simulink model "Hierarchical_control"  (R2023a)
settings: Solver=VariableStepAuto  StartTime=0.0  StopTime=T  RelTol=1e-3
InitFcn:
  | %% INITIALIZATION
  | run('LOAD_HIERARCHICAL.m');
  | %% UAV PARAMETERS
  | mass = 0.85;
  | Ib = diag([2.5 2.1 4.3])*10^-2;
  | %% SAMPLING TIME
  | Ts=0.01;
libraries: robotcorelib x1, uavutilslib x1
settings Model: Creator=salvatoregranata  LastModifiedBy=salvatoregranata

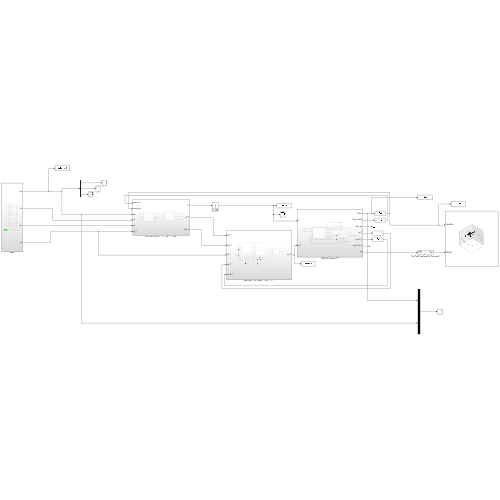
[thumbnail: Simulink's stored preview of the top-level diagram]
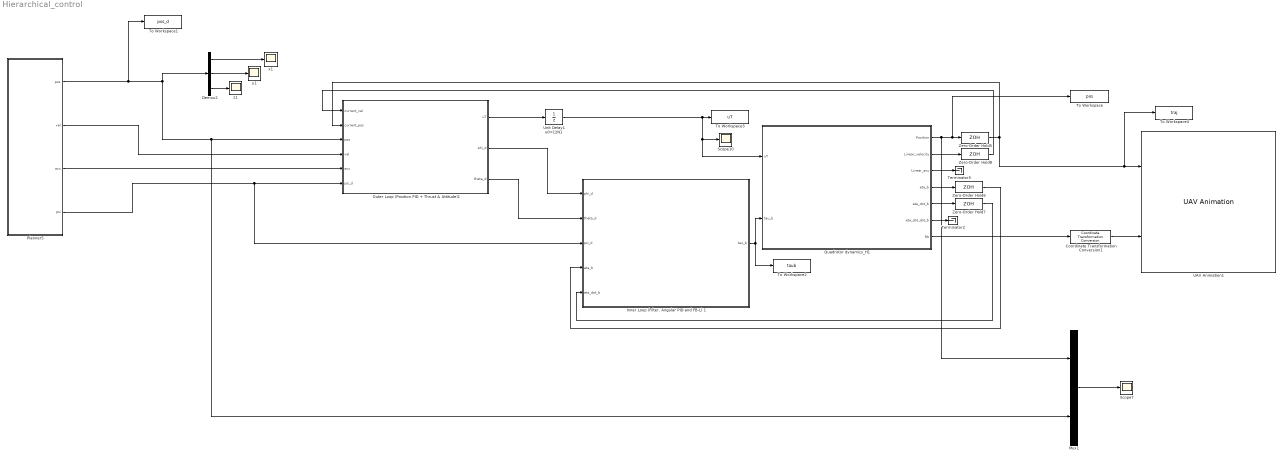
== system Hierarchical_control ==
  Coordinate Transformation Conversion1 : robotcorelib/Coordinate Transformation Conversion  InputRepresentation=Rotation Matrix  InputEulerSequence=ZYX  ShowTrVecInputPort=on  OutputRepresentation=Quaternion  OutputEulerSequence=ZYX  ShowTrVecOutputPort=on  SimulateUsing=Interpreted execution
  Demux2 : Demux  Outputs=3
  "Inner Loop (Filter, Angular PID and FB-L) 1" : Subsystem
  Mux1 : Mux  Inputs=2
  Outer Loop (Position PID + Thrust & Attitude)1 : Subsystem
  Planner5 : Subsystem
  Quadrotor dynamics_H1 : Subsystem
  Scope10 : Scope
  Scope7 : Scope
  Terminator2 : Terminator
  Terminator5 : Terminator
  To Workspace : ToWorkspace  VariableName=pos  SaveFormat=Structure With Time  SampleTime=-1
  To Workspace1 : ToWorkspace  VariableName=pos_d  SaveFormat=Structure With Time  SampleTime=-1
  To Workspace2 : ToWorkspace  VariableName=taub  SaveFormat=Structure With Time  SampleTime=-1
  To Workspace3 : ToWorkspace  VariableName=uT  SaveFormat=Structure With Time  SampleTime=-1
  To Workspace4 : ToWorkspace  VariableName=traj  SaveFormat=Structure With Time  SampleTime=-1
  UAV Animation1 : uavutilslib/UAV Animation  UAVType=Multirotor  UAVSize=1  InertialZDirection=Up  SampleTime=0.001
  Unit Delay1 u0=12N1 : UnitDelay  InitialCondition=11.772  SampleTime=Ts
  Zero-Order Hold{5..8} (4 alike) : ZeroOrderHold  SampleTime=Ts
  x1 : Scope
  y1 : Scope
  z1 : Scope
  wires:
  Coordinate Transformation Conversion1/1 -> UAV Animation1/2
  Quadrotor dynamics_H1/5(eta_dot_b) -> Zero-Order Hold7/1
  "Inner Loop (Filter, Angular PID and FB-L) 1"/1(tau_b) -> To Workspace2/1, Quadrotor dynamics_H1/2(tau_b)
  Planner5/3(acc) -> Outer Loop (Position PID + Thrust & Attitude)1/5(acc)
  Quadrotor dynamics_H1/6(eta_dot_dot_b) -> Terminator2/1
  Quadrotor dynamics_H1/2(Linear_velocity) -> Zero-Order Hold8/1
  Zero-Order Hold8/1 -> Outer Loop (Position PID + Thrust & Attitude)1/1(current_vel)
  Planner5/1(pos) -> To Workspace1/1, Mux1/2, Outer Loop (Position PID + Thrust & Attitude)1/3(pos), Demux2/1
  Mux1/1 -> Scope7/1
  Zero-Order Hold6/1 -> "Inner Loop (Filter, Angular PID and FB-L) 1"/4(eta_b)
  Outer Loop (Position PID + Thrust & Attitude)1/1(uT) -> Unit Delay1 u0=12N1/1
  Demux2/1 -> x1/1
  Zero-Order Hold7/1 -> "Inner Loop (Filter, Angular PID and FB-L) 1"/5(eta_dot_b)
  Planner5/4(psi) -> "Inner Loop (Filter, Angular PID and FB-L) 1"/3(psi_d), Outer Loop (Position PID + Thrust & Attitude)1/6(psi_d)
  Unit Delay1 u0=12N1/1 -> To Workspace3/1, Scope10/1, Quadrotor dynamics_H1/1(uT)
  Demux2/3 -> z1/1
  Demux2/2 -> y1/1
  Outer Loop (Position PID + Thrust & Attitude)1/3(theta_d) -> "Inner Loop (Filter, Angular PID and FB-L) 1"/2(theta_d)
  Quadrotor dynamics_H1/7(Rb) -> Coordinate Transformation Conversion1/1
  Quadrotor dynamics_H1/4(eta_b) -> Zero-Order Hold6/1
  Outer Loop (Position PID + Thrust & Attitude)1/2(phi_d) -> "Inner Loop (Filter, Angular PID and FB-L) 1"/1(phi_d)
  Quadrotor dynamics_H1/1(Position) -> Mux1/1, To Workspace/1, Zero-Order Hold5/1
  Quadrotor dynamics_H1/3(Linear_acc) -> Terminator5/1
  Planner5/2(vel) -> Outer Loop (Position PID + Thrust & Attitude)1/4(vel)
  Zero-Order Hold5/1 -> To Workspace4/1, UAV Animation1/1, Outer Loop (Position PID + Thrust & Attitude)1/2(current_pos)

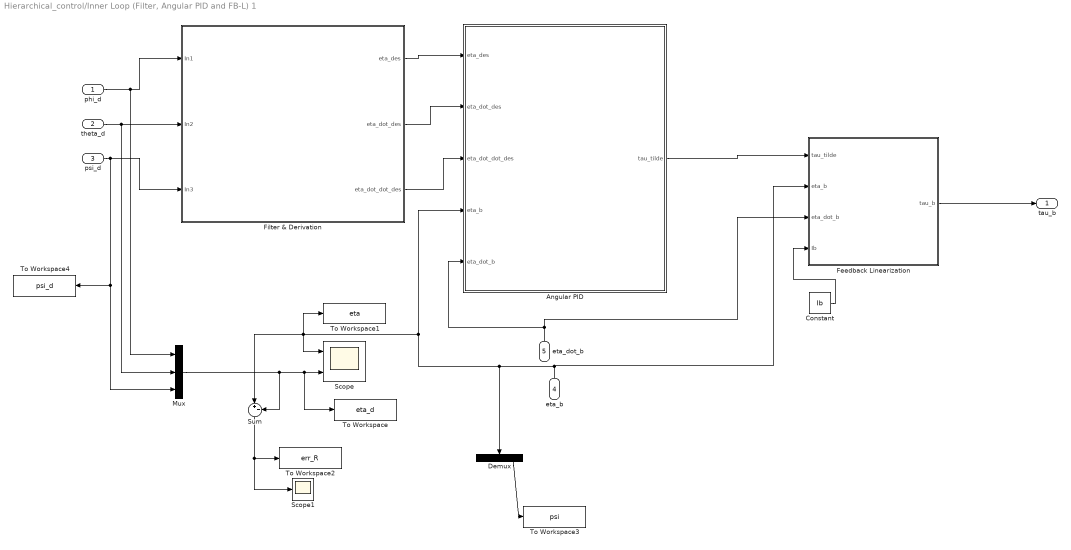
== system Hierarchical_control/Inner Loop (Filter, Angular PID and FB-L) 1 ==
  phi_d : Inport
  theta_d : Inport  Port=2
  psi_d : Inport  Port=3
  eta_b : Inport  Port=4
  eta_dot_b : Inport  Port=5
  Angular PID : MATLAB Function  TreatAsAtomicUnit=on
  Constant : Constant  Value=Ib
  Demux : Demux  Outputs=3
  Feedback Linearization : MATLAB Function  TreatAsAtomicUnit=on
  Filter & Derivation : Subsystem
  Mux : Mux  Inputs=3
  Scope : Scope  NumInputPorts=2
  Scope1 : Scope
  Sum : Sum  Inputs=|+-
  To Workspace : ToWorkspace  VariableName=eta_d  SaveFormat=Structure With Time  SampleTime=-1
  To Workspace1 : ToWorkspace  VariableName=eta  SaveFormat=Structure With Time  SampleTime=-1
  To Workspace2 : ToWorkspace  VariableName=err_R  SaveFormat=Structure With Time  SampleTime=-1
  To Workspace3 : ToWorkspace  VariableName=psi  SaveFormat=Structure With Time  SampleTime=-1
  To Workspace4 : ToWorkspace  VariableName=psi_d  SaveFormat=Structure With Time  SampleTime=-1
  tau_b : Outport
  wires:
  phi_d/1 -> Mux/1, Filter & Derivation/1(In1)
  theta_d/1 -> Mux/2, Filter & Derivation/2(In2)
  psi_d/1 -> Mux/3, To Workspace4/1, Filter & Derivation/3(In3)
  Filter & Derivation/1(eta_des) -> Angular PID/1(eta_des)
  Filter & Derivation/2(eta_dot_des) -> Angular PID/2(eta_dot_des)
  Filter & Derivation/3(eta_dot_dot_des) -> Angular PID/3(eta_dot_dot_des)
  Angular PID/1(tau_tilde) -> Feedback Linearization/1(tau_tilde)
  Feedback Linearization/1(tau_b) -> tau_b/1
  eta_b/1 -> Feedback Linearization/2(eta_b), Sum/1, Scope/1, To Workspace1/1, Angular PID/4(eta_b), Demux/1
  eta_dot_b/1 -> Angular PID/5(eta_dot_b), Feedback Linearization/3(eta_dot_b)
  Constant/1 -> Feedback Linearization/4(Ib)
  Mux/1 -> Sum/2, To Workspace/1, Scope/2
  Sum/1 -> Scope1/1, To Workspace2/1
  Demux/3 -> To Workspace3/1

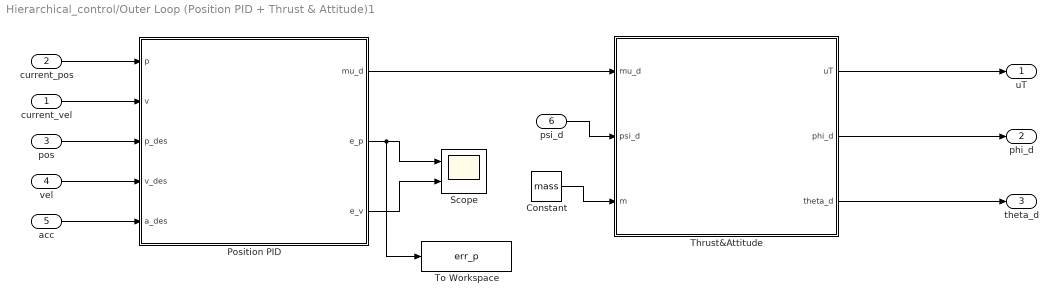
== system Hierarchical_control/Outer Loop (Position PID + Thrust & Attitude)1 ==
  current_vel : Inport
  current_pos : Inport  Port=2
  pos : Inport  Port=3
  vel : Inport  Port=4
  acc : Inport  Port=5
  psi_d : Inport  Port=6
  Constant : Constant  Value=mass
  Position PID : MATLAB Function  TreatAsAtomicUnit=on
  Scope : Scope  NumInputPorts=2
  Thrust&Attitude : MATLAB Function  TreatAsAtomicUnit=on
  To Workspace : ToWorkspace  VariableName=err_p  SaveFormat=Structure With Time  SampleTime=-1
  uT : Outport
  phi_d : Outport  Port=2
  theta_d : Outport  Port=3
  wires:
  pos/1 -> Position PID/3(p_des)
  vel/1 -> Position PID/4(v_des)
  acc/1 -> Position PID/5(a_des)
  Position PID/2(e_p) -> To Workspace/1, Scope/1
  Position PID/3(e_v) -> Scope/2
  Position PID/1(mu_d) -> Thrust&Attitude/1(mu_d)
  Thrust&Attitude/1(uT) -> uT/1
  Thrust&Attitude/2(phi_d) -> phi_d/1
  Thrust&Attitude/3(theta_d) -> theta_d/1
  psi_d/1 -> Thrust&Attitude/2(psi_d)
  current_pos/1 -> Position PID/1(p)
  current_vel/1 -> Position PID/2(v)
  Constant/1 -> Thrust&Attitude/3(m)

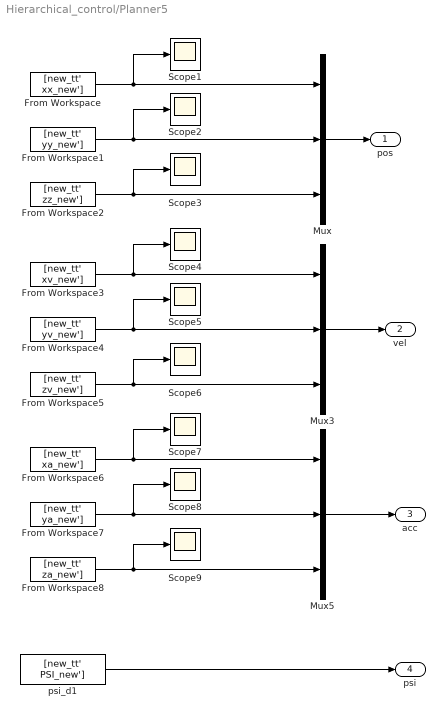
== system Hierarchical_control/Planner5 ==
  From Workspace : FromWorkspace  VariableName=[new_tt' xx_new']
  From Workspace1 : FromWorkspace  VariableName=[new_tt' yy_new']
  From Workspace2 : FromWorkspace  VariableName=[new_tt' zz_new']
  From Workspace3 : FromWorkspace  VariableName=[new_tt' xv_new']
  From Workspace4 : FromWorkspace  VariableName=[new_tt' yv_new']
  From Workspace5 : FromWorkspace  VariableName=[new_tt' zv_new']
  From Workspace6 : FromWorkspace  VariableName=[new_tt' xa_new']
  From Workspace7 : FromWorkspace  VariableName=[new_tt' ya_new']
  From Workspace8 : FromWorkspace  VariableName=[new_tt' za_new']
  Mux : Mux  Inputs=3
  Mux3 : Mux  Inputs=3
  Mux5 : Mux  Inputs=3
  Scope{1..9} (9 alike) : Scope
  psi_d1 : FromWorkspace  VariableName=[new_tt' PSI_new']  SampleTime=Ts
  pos : Outport
  vel : Outport  Port=2
  acc : Outport  Port=3
  psi : Outport  Port=4
  wires:
  Mux5/1 -> acc/1
  From Workspace1/1 -> Mux/2, Scope2/1
  Mux3/1 -> vel/1
  From Workspace6/1 -> Mux5/1, Scope7/1
  From Workspace2/1 -> Mux/3, Scope3/1
  From Workspace4/1 -> Mux3/2, Scope5/1
  Mux/1 -> pos/1
  From Workspace/1 -> Mux/1, Scope1/1
  From Workspace7/1 -> Mux5/2, Scope8/1
  From Workspace8/1 -> Scope9/1, Mux5/3
  From Workspace3/1 -> Mux3/1, Scope4/1
  From Workspace5/1 -> Mux3/3, Scope6/1
  psi_d1/1 -> psi/1

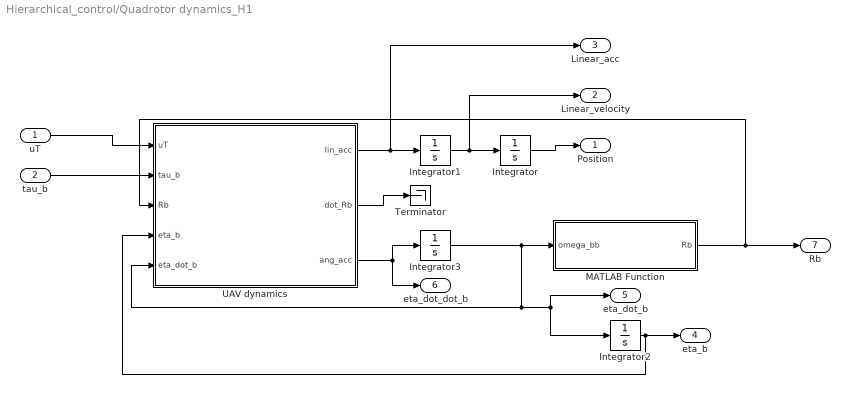
== system Hierarchical_control/Quadrotor dynamics_H1 ==
  uT : Inport
  tau_b : Inport  Port=2
  Integrator : Integrator  InitialCondition=[-1 -1.2 2]
  Integrator1 : Integrator  InitialCondition=[0 0 0]
  Integrator2 : Integrator  InitialCondition=[0 0 0]
  Integrator3 : Integrator  InitialCondition=[0 0 0]
  MATLAB Function : MATLAB Function  TreatAsAtomicUnit=on
  Terminator : Terminator
  UAV dynamics : MATLAB Function  TreatAsAtomicUnit=on
  Position : Outport
  Linear_velocity : Outport  Port=2
  Linear_acc : Outport  Port=3
  eta_b : Outport  Port=4
  eta_dot_b : Outport  Port=5
  eta_dot_dot_b : Outport  Port=6
  Rb : Outport  Port=7
  wires:
  tau_b/1 -> UAV dynamics/2(tau_b)
  Integrator/1 -> Position/1
  UAV dynamics/3(ang_acc) -> Integrator3/1, eta_dot_dot_b/1
  UAV dynamics/1(lin_acc) -> Linear_acc/1, Integrator1/1
  uT/1 -> UAV dynamics/1(uT)
  Integrator1/1 -> Linear_velocity/1, Integrator/1
  Integrator3/1 -> UAV dynamics/5(eta_dot_b), eta_dot_b/1, Integrator2/1, MATLAB Function/1(omega_bb)
  UAV dynamics/2(dot_Rb) -> Terminator/1
  MATLAB Function/1(Rb) -> Rb/1, UAV dynamics/3(Rb)
  Integrator2/1 -> UAV dynamics/4(eta_b), eta_b/1

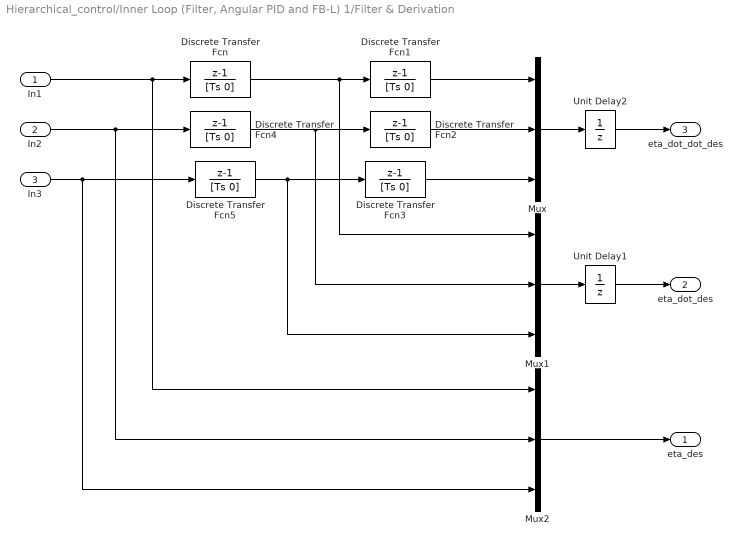
== system Hierarchical_control/Inner Loop (Filter, Angular PID and FB-L) 1/Filter & Derivation ==
  In1 : Inport
  In2 : Inport  Port=2
  In3 : Inport  Port=3
  Discrete Transfer Fcn{,1..5} (6 alike) : DiscreteTransferFcn  Numerator=[1 -1]  Denominator=[Ts 0]  SampleTime=Ts
  Mux : Mux  Inputs=3
  Mux1 : Mux  Inputs=3
  Mux2 : Mux  Inputs=3
  Unit Delay1 : UnitDelay  InitialCondition=[0 0 0]  SampleTime=Ts
  Unit Delay2 : UnitDelay  InitialCondition=[0 0 0]  SampleTime=Ts
  eta_des : Outport
  eta_dot_des : Outport  Port=2
  eta_dot_dot_des : Outport  Port=3
  wires:
  Discrete Transfer Fcn3/1 -> Mux/3
  Unit Delay1/1 -> eta_dot_des/1
  Discrete Transfer Fcn1/1 -> Mux/1
  In2/1 -> Discrete Transfer Fcn4/1, Mux2/2
  Unit Delay2/1 -> eta_dot_dot_des/1
  Discrete Transfer Fcn/1 -> Discrete Transfer Fcn1/1, Mux1/1
  Discrete Transfer Fcn2/1 -> Mux/2
  Discrete Transfer Fcn5/1 -> Mux1/3, Discrete Transfer Fcn3/1
  In3/1 -> Discrete Transfer Fcn5/1, Mux2/3
  Mux/1 -> Unit Delay2/1
  Discrete Transfer Fcn4/1 -> Discrete Transfer Fcn2/1, Mux1/2
  Mux2/1 -> eta_des/1
  Mux1/1 -> Unit Delay1/1
  In1/1 -> Discrete Transfer Fcn/1, Mux2/1

== matlab function Hierarchical_control/Inner Loop (Filter, Angular PID and FB-L) 1/Angular PID ==
  data: eta_des input; tau_tilde output; eta_dot_des input; eta_dot_dot_des input; eta_b input; eta_dot_b input
function tau_tilde = fcn(eta_des, eta_dot_des, eta_dot_dot_des, eta_b, eta_dot_b)

Ke=[diag([3 3 3]),diag([2 2 15])];

%compute the error
e_eta = eta_b-eta_des;
e_omega = eta_dot_b-eta_dot_des;
e=[e_eta;e_omega];

%simulate PD+
tau_tilde = -Ke*e + eta_dot_dot_des;

end

== matlab function Hierarchical_control/Inner Loop (Filter, Angular PID and FB-L) 1/Feedback Linearization ==
  data: tau_tilde input; tau_b output; eta_b input; eta_dot_b input; Ib input
function tau_b = fcn(tau_tilde,eta_b,eta_dot_b,Ib)

%inizialization
phi=eta_b(1);
theta=eta_b(2);
psi=eta_b(3);

phi_dot=eta_dot_b(1);
theta_dot=eta_dot_b(2);
psi_dot=eta_dot_b(3);

%definition trasformation matrix
Q=[1 ,     0      , -sin(theta);
   0 , cos(phi)   ,  cos(theta)*sin(phi);
   0 ,-sin(phi)   ,  cos(theta)*cos(phi)];

%definition the time derivative oftrasformation matrix
Q_dot=[0 ,     0            , -cos(theta)*theta_dot            ;
       0 , -sin(phi)*phi_dot,  cos(phi)*phi_dot*cos(theta)-sin(phi)*sin(theta)*theta_dot;
       0 , -cos(phi)*phi_dot, -sin(phi)*phi_dot*cos(theta)-cos(phi)*theta_dot*sin(theta)];

S=skew(Q*eta_dot_b);

C=Q'*S*Ib*Q+Q'*Ib*Q_dot;
tau_b  = Ib*Q*tau_tilde + inv(Q')*C*eta_dot_b;


%skew symmetric operator
function S = skew(v)
if(numel(v)~= 1)
S= [0 -v(3) v(2); 
    v(3) 0 -v(1);
    -v(2) v(1) 0];
else
S= zeros(3);
end

== matlab function Hierarchical_control/Outer Loop (Position PID + Thrust & Attitude)1/Position PID ==
  data: p input; mu_d output; v input; p_des input; v_des input; a_des input; e_p output; e_v output
function [mu_d,e_p,e_v] = fcn(p, v, p_des, v_des, a_des)

K = [diag([12 12 18]),diag([0.7 0.7 2.5])];  %Kp and Kv 

g=9.81;

%compute the error
e_p = p-p_des;
e_v = v-v_des;

e  = [e_p ; e_v];

mu_d = -K*e + a_des;


if(mu_d(3)>=g)
    display("singolarita'");
    mu_d(3) = 9.8;
end

== matlab function Hierarchical_control/Outer Loop (Position PID + Thrust & Attitude)1/Thrust&Attitude ==
  data: mu_d input; uT output; psi_d input; phi_d output; theta_d output; m input
function [uT,phi_d,theta_d] = fcn(mu_d,psi_d,m)
g=9.81;

%compute the thrust
uT = m*sqrt(mu_d(1)^2 + mu_d(2)^2 + (mu_d(3) - g)^2);

%compute the attitude
phi_d = asin((m/uT)* (mu_d(2)*cos(psi_d)- mu_d(1)*sin(psi_d)) );       %desired roll

theta_d = atan((mu_d(1)*cos(psi_d)+mu_d(2)*sin(psi_d))/(mu_d(3)-g));     %desired pitch

end

== matlab function Hierarchical_control/Quadrotor dynamics_H1/MATLAB Function ==
  data: omega_bb input; Rb output
function Rb = fcn(omega_bb)

Rb = expm(skew(omega_bb));
end

function S = skew(v)
if(numel(v)~= 1)
S= [0 -v(3) v(2); 
    v(3) 0 -v(1);
    -v(2) v(1) 0];
else
S= zeros(3);
end
end

== matlab function Hierarchical_control/Quadrotor dynamics_H1/UAV dynamics ==
  data: uT input size=1; tau_b input size=3; lin_acc output size=3; Rb input size=[3,3]; eta_b input; eta_dot_b input size=3; dot_Rb output size=[3,3]; ang_acc output size=3; mass parameter size=1; Ib parameter size=[3,3]
function [lin_acc, dot_Rb, ang_acc] = fcn(uT,tau_b,Rb,eta_b, eta_dot_b,mass, Ib)

phi=eta_b(1);
theta=eta_b(2);
phi_dot=eta_dot_b(1);
theta_dot=eta_dot_b(2);

Q=[1 ,     0      , -sin(theta);
   0 , cos(phi)   ,  cos(theta)*sin(phi);
   0 ,-sin(phi)   ,  cos(theta)*cos(phi)];

Q_dot=[0 ,     0            , -cos(theta)*theta_dot            ;
       0 , -sin(phi)*phi_dot,  cos(phi)*phi_dot*cos(theta)-sin(phi)*sin(theta)*theta_dot;
       0 , -cos(phi)*phi_dot, -sin(phi)*phi_dot*cos(theta)-cos(phi)*theta_dot*sin(theta)];

S=skew(Q*eta_dot_b);

C=Q'*S*Ib*Q+Q'*Ib*Q_dot;
M=Q'*Ib*Q;

lin_acc = 9.81*[0 0 1]'-(uT/mass)*Rb*[0 0 1]';
dot_Rb = Rb*skew(eta_dot_b);
ang_acc = M\(-C*eta_dot_b + Q'*tau_b);

end

function S = skew(v)
if(numel(v)~= 1)
S= [0 -v(3) v(2); 
    v(3) 0 -v(1);
    -v(2) v(1) 0];
else
S= zeros(3);
end
end
